simulink library "Turbine_State_Machine_Lib"  (R2026a)
settings: Solver=ode45  EnableMultiTasking=on
Description:
  | Copyright 2009-2026 The MathWorks, Inc. MathWorks, Inc.
settings Model: Creator=smiller  LastModifiedBy=smiller
settings DataIOCC: SignalLoggingSaveFormat=ModelDataLogs
settings DebuggingCC: UnderspecifiedInitializationDetection=Classic  PregeneratedLibrarySubsystemCodeDiagnostic=none
settings HardwareCC: ProdHWDeviceType=32-bit Generic
settings GRTTargetCC: CombineOutputUpdateFcns=off  GRTInterface=on

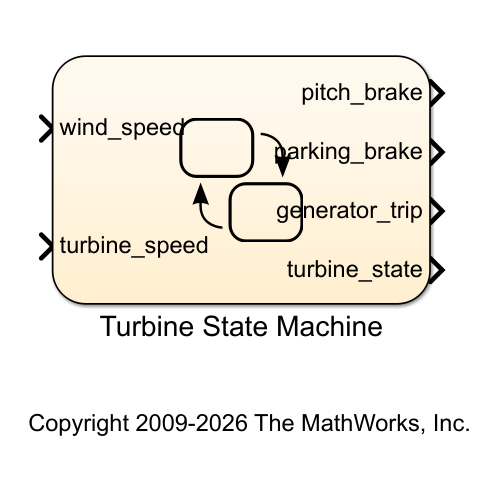
[thumbnail: Simulink's stored preview of the top-level diagram]
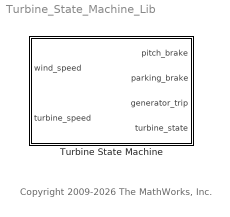
== system Turbine_State_Machine_Lib ==
  note: Copyright 2009-2026 The MathWorks, Inc.
  Turbine State Machine : Stateflow chart  TreatAsAtomicUnit=on

== stateflow chart Turbine_State_Machine_Lib/Turbine State Machine ==
  state Generating
    entry: parking_brake = 0;
    generator_trip = 0;
    pitch_brake = 0;
    turbine_state = 2;
  state Startup
    entry: parking_brake = 0;
    generator_trip = 1;
    pitch_brake = 0;
    turbine_state = 1;
  state Park
    entry: parking_brake = 1;
    generator_trip = 1;
    pitch_brake = 1;
    turbine_state = 0;
  state Brake
    entry: parking_brake = 0;
    generator_trip = 1;
    pitch_brake = 1;
    turbine_state = 3;
  Startup -> Generating [order 1] : [turbine_speed>...
      | turbine_speed_cut_in]
  Park -> Startup : [wind_speed>...
      | wind_speed_cut_in_lower...
      | &&wind_speed<...
      | wind_speed_cut_out]
  Startup -> Brake [order 2] : [wind_speed<...
      | wind_speed_cut_in_lower]
  Brake -> Startup [order 2] : [wind_speed<...
      | wind_speed_cut_in_upper...
      | && wind_speed>...
      | wind_speed_cut_in_lower]
  Generating -> Brake : [wind_speed<...
      | wind_speed_cut_in_lower...
      | ||wind_speed>...
      | wind_speed_cut_out...
      | ||turbine_speed>...
      | turbine_speed_cut_out...
      | ||turbine_speed<...
      | turbine_speed_cut_in*0.9]
  (default) -> Park
  Brake -> Park [order 1] : [turbine_speed<=...
      | park_speed]
  data: pitch_brake output double; wind_speed input; turbine_speed input; parking_brake output double; generator_trip output double; wind_speed_cut_in_lower local double =WT_Params.Main_Controller.wind_speed_cut_in_lower; turbine_speed_cut_in local double =WT_Params.Main_Controller.turbine_speed_cut_in; turbine_state output double; wind_speed_cut_out local double =WT_Params.Main_Controller.wind_speed_cut_out; wind_speed_cut_in_upper local double =WT_Params.Main_Controller.wind_speed_cut_in_upper; turbine_speed_cut_out local double =WT_Params.Main_Controller.turbine_speed_cut_out; park_speed constant double =WT_Params.Main_Controller.turbine_speed_park
